simulink model "two_gen_model_2020b"  (R2020b)
settings: Solver=VariableStepAuto  StartTime=0.0  StopTime=t_final  MaxStep=t_max_step  RelTol=1e-3
values from neighbouring files (symbols this model uses):
  a_21 = (12e3)^2 * abs(1 / (1j * ws * 0.0275))    [main.m]    (also in main_one_gen.m; main_two_gen.m)
  D1 = 0.18 * K1    (= 1.5714e-08)    [main_two_gen.m]
  D2 = 0.18 * K1    (= 1.5714e-08)    [main_two_gen.m]
  d2_0 = d2_0_array(ii)    [main_two_gen.m]
  K1 = 8.73e-8    (= 8.73e-08)    [main_two_gen.m]
  K2 = 6.12e-8    (= 6.12e-08)    [main_two_gen.m]
  P1_ref = 1e6    (= 1000000)    [main_two_gen.m]
  P2_ref = 1e6    (= 1000000)    [main_two_gen.m]
  w1_0 = w1_array(ij)    [main_two_gen.m]
  w2_0 = w2_array(ik)    [main_two_gen.m]
  ws = 50 * 2 * pi    (= 314.159265359)    [main.m]    (also in main_one_gen.m; main_two_gen.m)
settings Model: Creator=Liraz  LastModifiedBy=Liraz
settings DebuggingCC: UnconnectedInputMsg=none  UnconnectedOutputMsg=none  UnconnectedLineMsg=none  SFMachineParentedDataDiag=error

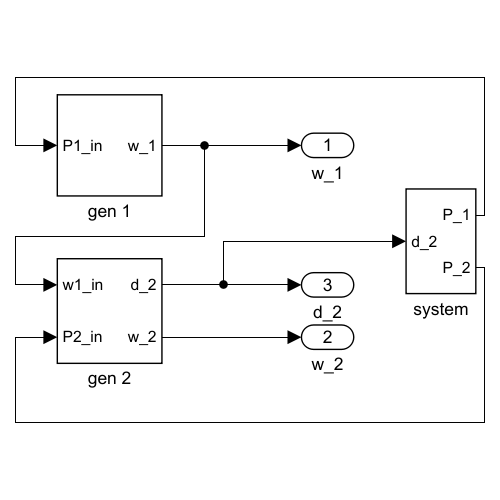
[thumbnail: Simulink's stored preview of the top-level diagram]
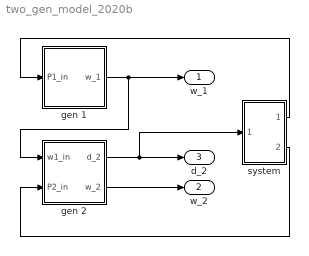
== system two_gen_model_2020b ==
  gen 1 : Subsystem
  gen 2 : Subsystem
  system : Subsystem
  w_1 : Outport
  w_2 : Outport  Port=2
  d_2 : Outport  Port=3
  wires:
  system/1(P_1) -> gen 1/1(P1_in)
  system/2(P_2) -> gen 2/2(P2_in)
  gen 1/1(w_1) -> w_1/1, gen 2/1(w1_in)
  gen 2/1(d_2) -> system/1(d_2), d_2/1
  gen 2/2(w_2) -> w_2/1

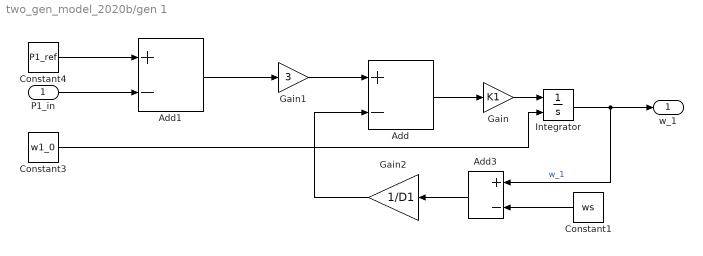
== system two_gen_model_2020b/gen 1 ==
  P1_in : Inport
  Add : Sum  Inputs=+-
  Add1 : Sum  Inputs=+-
  Add3 : Sum  Inputs=+-
  Constant1 : Constant  Value=ws
  Constant3 : Constant  Value=w1_0
  Constant4 : Constant  Value=P1_ref
  Gain : Gain  Gain=K1
  Gain1 : Gain  Gain=3
  Gain2 : Gain  Gain=1/D1
  Integrator : Integrator  InitialConditionSource=external
  w_1 : Outport
  wires:
  Constant4/1 -> Add1/1
  Constant3/1 -> Integrator/2
  Add1/1 -> Gain1/1
  Add/1 -> Gain/1
  Add3/1 -> Gain2/1
  Gain/1 -> Integrator/1
  Integrator/1 -> w_1/1, Add3/1  "w_1"
  P1_in/1 -> Add1/2
  Gain1/1 -> Add/1
  Constant1/1 -> Add3/2
  Gain2/1 -> Add/2

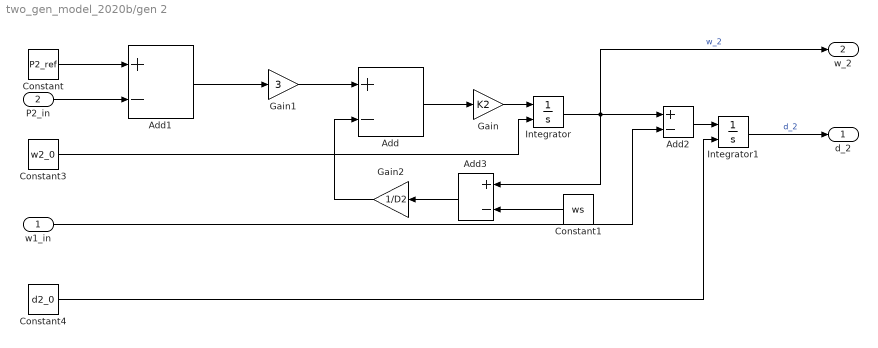
== system two_gen_model_2020b/gen 2 ==
  w1_in : Inport
  P2_in : Inport  Port=2
  Add{,1..3} (4 alike) : Sum  Inputs=+-
  Constant : Constant  Value=P2_ref
  Constant1 : Constant  Value=ws
  Constant3 : Constant  Value=w2_0
  Constant4 : Constant  Value=d2_0
  Gain : Gain  Gain=K2
  Gain1 : Gain  Gain=3
  Gain2 : Gain  Gain=1/D2
  Integrator : Integrator  InitialConditionSource=external
  Integrator1 : Integrator  InitialConditionSource=external
  d_2 : Outport
  w_2 : Outport  Port=2
  wires:
  w1_in/1 -> Add2/2
  Constant4/1 -> Integrator1/2
  Gain/1 -> Integrator/1
  Integrator/1 -> Add3/1, w_2/1, Add2/1  "w_2"
  Add1/1 -> Gain1/1
  Gain1/1 -> Add/1
  Add2/1 -> Integrator1/1
  Gain2/1 -> Add/2
  P2_in/1 -> Add1/2
  Constant3/1 -> Integrator/2
  Constant/1 -> Add1/1
  Add/1 -> Gain/1
  Integrator1/1 -> d_2/1  "d_2"
  Constant1/1 -> Add3/2
  Add3/1 -> Gain2/1

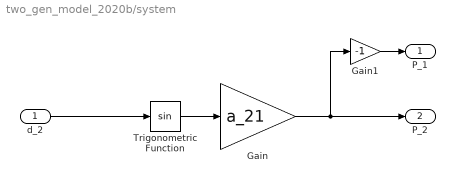
== system two_gen_model_2020b/system ==
  d_2 : Inport
  Gain : Gain  Gain=a_21
  Gain1 : Gain  Gain=-1
  Trigonometric Function : Trigonometry
  P_1 : Outport
  P_2 : Outport  Port=2
  wires:
  Gain/1 -> P_2/1, Gain1/1
  Trigonometric Function/1 -> Gain/1
  Gain1/1 -> P_1/1
  d_2/1 -> Trigonometric Function/1
